simulink model "F16_nonlinear_simulation_R2018b"  (R2018b)
settings: Solver=VariableStepAuto  StartTime=0.0  StopTime=60  MaxStep=1.2  RelTol=1e-3
libraries: simulink x5, aerolibutil x2, aerolibanimutils x1, vrlib x1
settings Model: Creator=parth  LastModifiedBy=parth
settings DataIOCC: ReturnWorkspaceOutputs=on

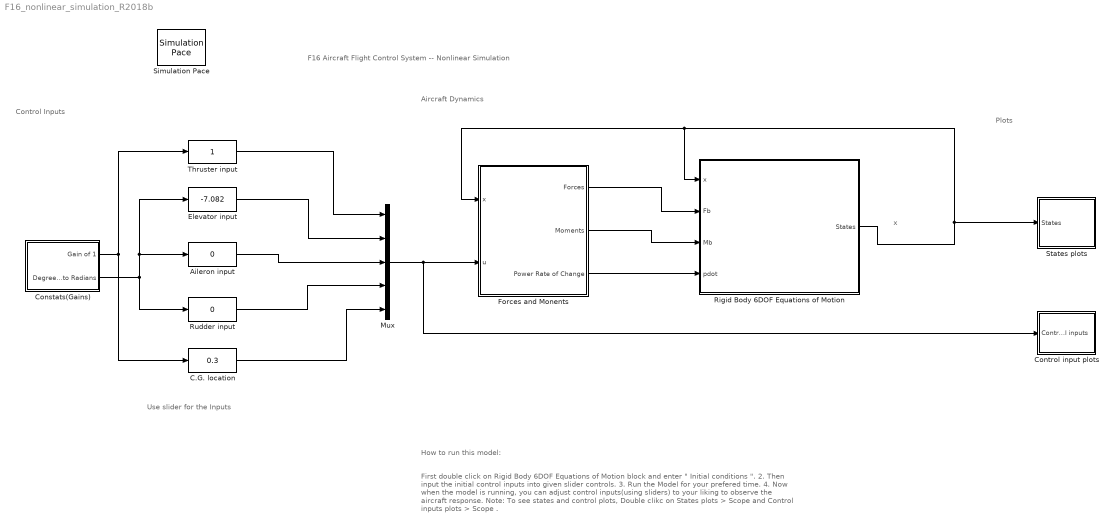
== system F16_nonlinear_simulation_R2018b ==
  note: x
  note: Plots
  note: Use slider for the Inputs
  note: F16 Aircraft Flight Control System -- Nonlinear Simulation
  note: Control Inputs
  note: Aircraft Dynamics
  note: First double click on Rigid Body 6DOF Equations of Motion block and enter " Initial conditions ".
      | 2. Then input the initial control inputs into given slider controls.
      | 3. Run the Model for your prefered time.
      | 4. Now when the model is running, you can adjust control inputs(using sliders) to your liking to observe the aircraft response.
      |
      | Note: To see states and control plots, Double clikc on States plots > Scope and Control inputs plots > Scope .
  note: How to run this model:
  Aileron input : simulink/Math Operations/Slider Gain  gain=0  low=-21.5  high=21.5
  C.G. location : simulink/Math Operations/Slider Gain  gain=0.3  low=0.3  high=0.4
  Constats(Gains) : Subsystem
  Control input plots : Subsystem
  Elevator input : simulink/Math Operations/Slider Gain  gain=-7.082  low=-25  high=25
  Forces and Monents : Subsystem
  Mux : Mux  Inputs=5
  "Rigid Body 6DOF Equations of Motion " : Subsystem  mask{V_init=502, alpha_init=0.3006, beta_init=0, p_init=0, q_init=0.3, r_init=0, phi_init=0, theta_init=0.3006, psi_init=0, Xe_init=0, Ye_init=0, h_init=1000, actual_power_init=90.566}
      mask prompts: V_init "V_init (ft/sec)"; alpha_init "alpha_init (rad)"; beta_init "beta_init (rad)"; p_init "p_init (rad/sec)"; q_init "q_init (rad/sec)"; r_init "r_init (rad/sec)"; phi_init "phi_init (rad)"; theta_init "theta_init (rad)"; psi_init "psi_init (rad)"; Xe_init "Xe_init (ft)"; Ye_init "Ye_init (ft)"; h_init "h_init (ft)"
      mask DialogControl ParameterGroupVar Prompt: Enter Aircraft Initial States here:
  Rudder input : simulink/Math Operations/Slider Gain  gain=0  low=-30  high=30
  Simulation Pace : aerolibanimutils/Simulation Pace  SimulationPace=1  SleepMode=Auto  OutputPaceError=off  SampleTime=1/30
  States plots : Subsystem
  Thruster input : simulink/Math Operations/Slider Gain  gain=1  low=0  high=1
  wires:
  Mux/1 -> Control input plots/1(Control inputs), Forces and Monents/2(u)
  Thruster input/1 -> Mux/1
  Elevator input/1 -> Mux/2
  Aileron input/1 -> Mux/3
  Forces and Monents/3(Power Rate of Change) -> "Rigid Body 6DOF Equations of Motion "/4(pdot)
  Constats(Gains)/1(Gain of 1) -> C.G. location/1, Thruster input/1
  Forces and Monents/1(Forces) -> "Rigid Body 6DOF Equations of Motion "/2(Fb)
  Forces and Monents/2(Moments) -> "Rigid Body 6DOF Equations of Motion "/3(Mb)
  Rudder input/1 -> Mux/4
  Constats(Gains)/2(Degree to Radians) -> Elevator input/1, Aileron input/1, Rudder input/1
  "Rigid Body 6DOF Equations of Motion "/1(States) -> Forces and Monents/1(x), "Rigid Body 6DOF Equations of Motion "/1(x), States plots/1(States)
  C.G. location/1 -> Mux/5

== system F16_nonlinear_simulation_R2018b/Constats(Gains) ==
  Constant(Gain) : Constant
  Degrees to Rad : Constant  Value=0.0175
  Gain of 1 : Outport
  Degree to Radians : Outport  Port=2
  wires:
  Degrees to Rad/1 -> Degree to Radians/1
  Constant(Gain)/1 -> Gain of 1/1

== system F16_nonlinear_simulation_R2018b/Control input plots ==
  Control inputs : Inport
  Demux : Demux
  Scope : Scope  NumInputPorts=4
  wires:
  Demux/4 -> Scope/4  "rudder"
  Demux/1 -> Scope/1  "throttle"
  Demux/3 -> Scope/3  "aileron"
  Control inputs/1 -> Demux/1
  Demux/2 -> Scope/2  "elevator"

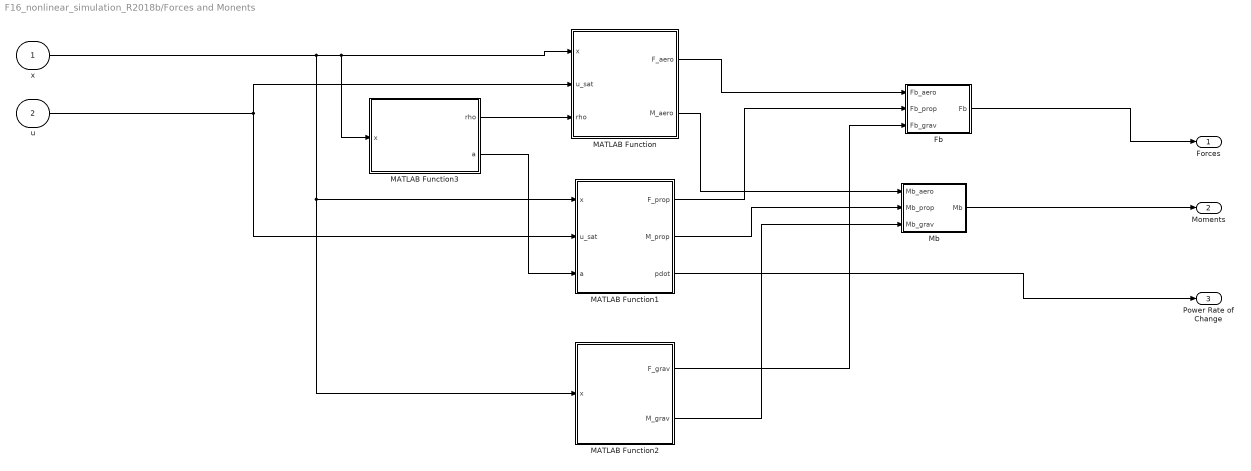
== system F16_nonlinear_simulation_R2018b/Forces and Monents ==
  x : Inport
  u : Inport  Port=2
  Fb : Subsystem
  MATLAB Function : MATLAB Function  TreatAsAtomicUnit=on
  MATLAB Function1 : MATLAB Function  TreatAsAtomicUnit=on
  MATLAB Function2 : MATLAB Function  TreatAsAtomicUnit=on
  MATLAB Function3 : MATLAB Function  TreatAsAtomicUnit=on
  Mb : Subsystem
  Forces : Outport
  Moments : Outport  Port=2
  Power Rate of Change : Outport  Port=3
  wires:
  Mb/1(Mb) -> Moments/1
  Fb/1(Fb) -> Forces/1
  x/1 -> MATLAB Function2/1(x), MATLAB Function1/1(x), MATLAB Function3/1(x), MATLAB Function/1(x)
  u/1 -> MATLAB Function1/2(u_sat), MATLAB Function/2(u_sat)
  MATLAB Function/1(F_aero) -> Fb/1(Fb_aero)
  MATLAB Function1/1(F_prop) -> Fb/2(Fb_prop)
  MATLAB Function2/1(F_grav) -> Fb/3(Fb_grav)
  MATLAB Function2/2(M_grav) -> Mb/3(Mb_grav)
  MATLAB Function1/2(M_prop) -> Mb/2(Mb_prop)
  MATLAB Function/2(M_aero) -> Mb/1(Mb_aero)
  MATLAB Function1/3(pdot) -> Power Rate of Change/1
  MATLAB Function3/1(rho) -> MATLAB Function/3(rho)
  MATLAB Function3/2(a) -> MATLAB Function1/3(a)

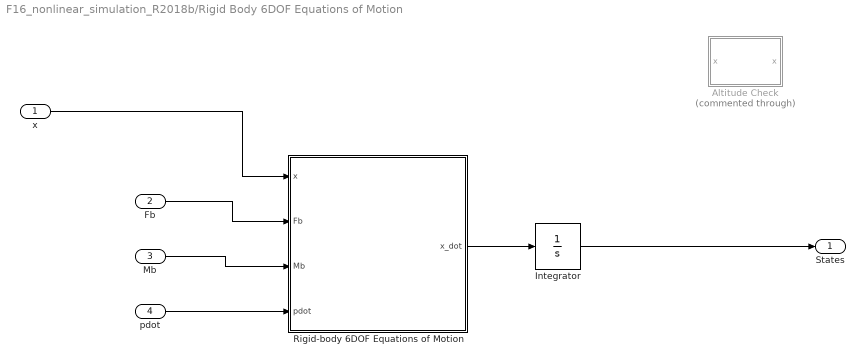
== system F16_nonlinear_simulation_R2018b/Rigid Body 6DOF Equations of Motion  ==
  x : Inport
  Fb : Inport  Port=2
  Mb : Inport  Port=3
  pdot : Inport  Port=4
  Altitude Check : MATLAB Function  Commented=through  TreatAsAtomicUnit=on
  Integrator : Integrator  InitialCondition=[(V_init*cos(alpha_init)*cos(beta_init)); (V_init*sin(beta_init)); (V_init*sin(alpha_init)*cos(beta_init)); p_init; q_init; r_init; phi_init; theta_init; psi_init; Xe_init; Ye_init; h_init; actual_power_init]
  Rigid-body 6DOF Equations of Motion : MATLAB Function  TreatAsAtomicUnit=on
  States : Outport
  wires:
  Fb/1 -> Rigid-body 6DOF Equations of Motion/2(Fb)
  x/1 -> Rigid-body 6DOF Equations of Motion/1(x)
  Rigid-body 6DOF Equations of Motion/1(x_dot) -> Integrator/1
  pdot/1 -> Rigid-body 6DOF Equations of Motion/4(pdot)
  Mb/1 -> Rigid-body 6DOF Equations of Motion/3(Mb)
  Integrator/1 -> States/1

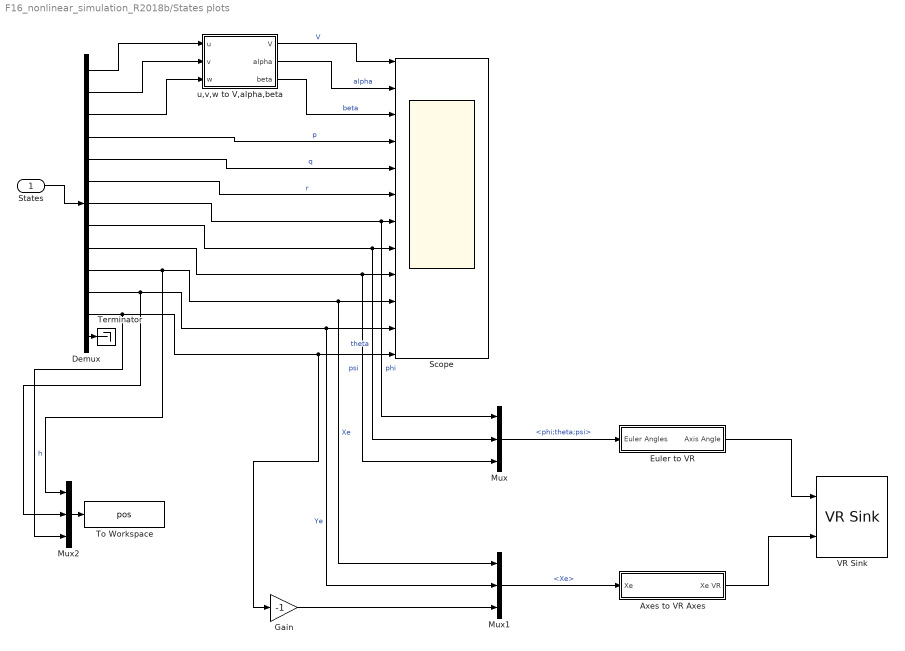
== system F16_nonlinear_simulation_R2018b/States plots ==
  States : Inport
  Axes to VR Axes : Subsystem
  Demux : Demux  Outputs=13
  Euler to VR : Subsystem
  Gain : Gain  Gain=-1
  Mux : Mux  Inputs=3
  Mux1 : Mux  Inputs=3
  Mux2 : Mux  Inputs=3
  Scope : Scope  NumInputPorts=12
  Terminator : Terminator
  To Workspace : ToWorkspace  VariableName=pos  SaveFormat=Timeseries  SampleTime=-1
  VR Sink : vrlib/VR Sink  InstantiateOnLoad=on  SampleTime=0.1  ViewEnable=on  RemoteChange=off  RemoteView=off  FieldsWritten=HL20.rotation.4.1.1.double#HL20.translation.3.1.1.double  WorldFileName=aeroblk_HL20.wrl  WorldDescription=aeroblk_HL20  AutoView=on  VideoDimensions=[]  AllowVariableSize=off  FigureProperties="{'Position', 'Name', 'Viewpoint', 'CameraBound', 'CameraDirection', 'CameraPosition', 'CameraUpVector', 'ZoomFactor', 'Antialiasing', 'Headlight', 'Lighting', 'NavPanel', 'Sound', 'StatusBar', 'Stereo3D', 'Stereo3DCameraOffset', 'Stereo3DHIT', 'ToolBar', 'Textures', 'Transparency', 'Triad', 'Wireframe', 'NavZones', 'NavMode', 'NavSpeed', 'CaptureFileFormat', 'CaptureFileName', 'Record2DCompressMethod', 'Record2DCompressQuality', 'Record2D', 'Record2DFileName', 'Record2DFPS'; [1.0000000000000000e+00   1.1800000000000000e+02   9.6000000000000000e+02   9.1100000000000000e+02], 'aeroblk_HL20', 'Rear Position', 'on', [-5.6194269145227393e-01  -1.3939411374335573e-04  -8.2717615541833223e-01], [1.4519874663616713e+02  -1.1012134985725118e-01   3.0148878051148063e+02], [4.0022421463915296e-03   9.9998782229421512e-01  -2.8874419604393194e-03], [1.0000000000000000e+00], 'on', 'on', 'on', 'halfbar', 'on', 'on', 'off', [1.0000000149011612e-01], [0.0000000000000000e+00], 'on', 'on', 'on', 'none', 'off', 'off', 'examine', 'normal', 'tif', '%f_anim_%n.tif', 'auto', [7.5000000000000000e+01], 'off', '%f_anim_%n.avi', 'auto'}"
  u,v,w to V,alpha,beta : MATLAB Function  TreatAsAtomicUnit=on
  wires:
  Demux/7 -> Mux/1, Scope/7  "phi"
  Demux/4 -> Scope/4  "p"
  Demux/13 -> Terminator/1
  Demux/1 -> u,v,w to V,alpha,beta/1(u)
  Demux/11 -> Mux2/2, Mux1/2, Scope/11  "Ye"
  Demux/3 -> u,v,w to V,alpha,beta/3(w)
  Demux/5 -> Scope/5  "q"
  States/1 -> Demux/1
  Demux/12 -> Mux2/3, Gain/1, Scope/12  "h"
  Demux/10 -> Mux2/1, Mux1/1, Scope/10  "Xe"
  Demux/2 -> u,v,w to V,alpha,beta/2(v)
  Demux/8 -> Mux/2, Scope/8  "theta"
  Demux/6 -> Scope/6  "r"
  Demux/9 -> Mux/3, Scope/9  "psi"
  u,v,w to V,alpha,beta/3(beta) -> Scope/3  "beta"
  u,v,w to V,alpha,beta/2(alpha) -> Scope/2  "alpha"
  u,v,w to V,alpha,beta/1(V) -> Scope/1  "V"
  Euler to VR/1(Axis Angle) -> VR Sink/1
  Mux/1 -> Euler to VR/1(Euler Angles)  "<phi;theta;psi>"
  Axes to VR Axes/1(Xe VR) -> VR Sink/2
  Mux1/1 -> Axes to VR Axes/1(Xe)  "<Xe>"
  Gain/1 -> Mux1/3
  Mux2/1 -> To Workspace/1

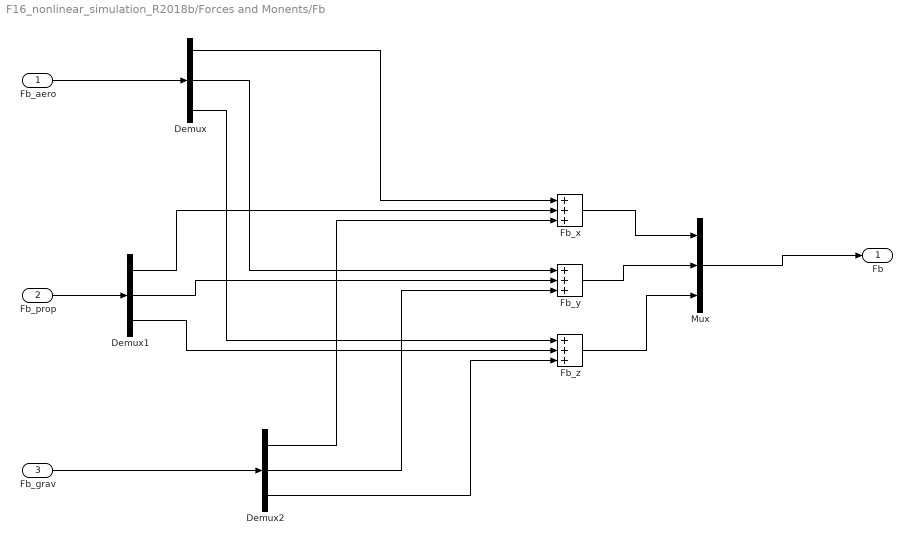
== system F16_nonlinear_simulation_R2018b/Forces and Monents/Fb ==
  Fb_aero : Inport
  Fb_prop : Inport  Port=2
  Fb_grav : Inport  Port=3
  Demux : Demux  Outputs=3
  Demux1 : Demux  Outputs=3
  Demux2 : Demux  Outputs=3
  Fb_x : Sum  Inputs=+++
  Fb_y : Sum  Inputs=+++
  Fb_z : Sum  Inputs=+++
  Mux : Mux  Inputs=3
  Fb : Outport
  wires:
  Demux1/2 -> Fb_y/2
  Demux/2 -> Fb_y/1
  Fb_x/1 -> Mux/1
  Demux/3 -> Fb_z/1
  Demux1/3 -> Fb_z/2
  Demux2/3 -> Fb_z/3
  Fb_z/1 -> Mux/3
  Demux1/1 -> Fb_x/2
  Demux2/1 -> Fb_x/3
  Fb_y/1 -> Mux/2
  Demux2/2 -> Fb_y/3
  Demux/1 -> Fb_x/1
  Mux/1 -> Fb/1
  Fb_aero/1 -> Demux/1
  Fb_prop/1 -> Demux1/1
  Fb_grav/1 -> Demux2/1

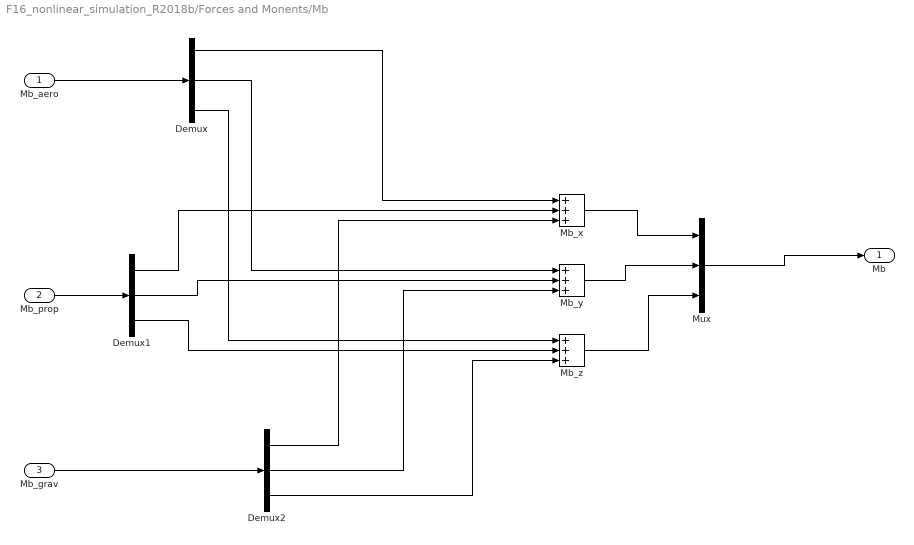
== system F16_nonlinear_simulation_R2018b/Forces and Monents/Mb ==
  Mb_aero : Inport
  Mb_prop : Inport  Port=2
  Mb_grav : Inport  Port=3
  Demux : Demux  Outputs=3
  Demux1 : Demux  Outputs=3
  Demux2 : Demux  Outputs=3
  Mb_x : Sum  Inputs=+++
  Mb_y : Sum  Inputs=+++
  Mb_z : Sum  Inputs=+++
  Mux : Mux  Inputs=3
  Mb : Outport
  wires:
  Demux1/2 -> Mb_y/2
  Demux/2 -> Mb_y/1
  Mb_x/1 -> Mux/1
  Demux/3 -> Mb_z/1
  Demux1/3 -> Mb_z/2
  Demux2/3 -> Mb_z/3
  Mb_z/1 -> Mux/3
  Demux1/1 -> Mb_x/2
  Demux2/1 -> Mb_x/3
  Mb_y/1 -> Mux/2
  Demux2/2 -> Mb_y/3
  Demux/1 -> Mb_x/1
  Mux/1 -> Mb/1
  Mb_aero/1 -> Demux/1
  Mb_prop/1 -> Demux1/1
  Mb_grav/1 -> Demux2/1

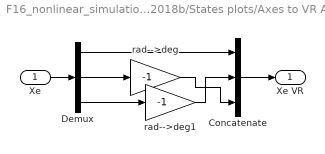
== system F16_nonlinear_simulation_R2018b/States plots/Axes to VR Axes ==
  Xe : Inport
  Concatenate : Concatenate  NumInputs=3
  Demux : Demux  Outputs=3
      settings: DisplayOption=none
  rad-->deg : Gain  Gain=-1  SaturateOnIntegerOverflow=on  OutDataTypeStr=Inherit: Same as input  ParamDataTypeStr=Inherit: Same as input
  rad-->deg1 : Gain  Gain=-1  SaturateOnIntegerOverflow=on  OutDataTypeStr=Inherit: Same as input  ParamDataTypeStr=Inherit: Same as input
  Xe VR : Outport  VectorParamsAs1DForOutWhenUnconnected=off
  wires:
  Xe/1 -> Demux/1
  Demux/1 -> Concatenate/1
  Demux/2 -> rad-->deg/1
  Demux/3 -> rad-->deg1/1
  Concatenate/1 -> Xe VR/1
  rad-->deg1/1 -> Concatenate/2
  rad-->deg/1 -> Concatenate/3

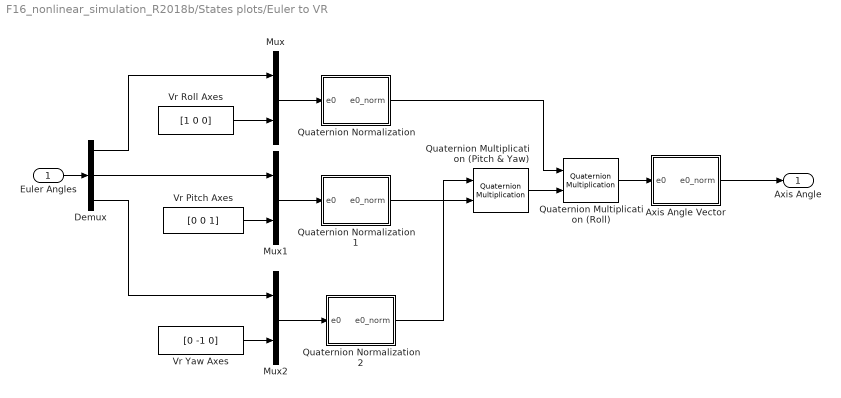
== system F16_nonlinear_simulation_R2018b/States plots/Euler to VR ==
  Euler Angles : Inport
  Axis Angle Vector : Subsystem
  Demux : Demux  Outputs=3
      settings: DisplayOption=none
  Mux : Mux  Inputs=2
  Mux1 : Mux  Inputs=2
  Mux2 : Mux  Inputs=2
  Quaternion Multiplication (Pitch & Yaw) : aerolibutil/Quaternion Multiplication
  Quaternion Multiplication (Roll) : aerolibutil/Quaternion Multiplication
  Quaternion Normalization : Subsystem
  Quaternion Normalization1 : Subsystem
  Quaternion Normalization2 : Subsystem
  Vr Pitch Axes : Constant  Value=[0 0 1]
  Vr Roll Axes : Constant  Value=[1 0 0]
  Vr Yaw Axes : Constant  Value=[0 -1 0]
  Axis Angle : Outport  VectorParamsAs1DForOutWhenUnconnected=off
  wires:
  Quaternion Multiplication (Roll)/1 -> Axis Angle Vector/1(e0)
  Quaternion Multiplication (Pitch & Yaw)/1 -> Quaternion Multiplication (Roll)/2
  Axis Angle Vector/1(e0_norm) -> Axis Angle/1
  Quaternion Normalization/1(e0_norm) -> Quaternion Multiplication (Roll)/1
  Quaternion Normalization2/1(e0_norm) -> Quaternion Multiplication (Pitch & Yaw)/1
  Quaternion Normalization1/1(e0_norm) -> Quaternion Multiplication (Pitch & Yaw)/2
  Mux2/1 -> Quaternion Normalization2/1(e0)
  Mux1/1 -> Quaternion Normalization1/1(e0)
  Mux/1 -> Quaternion Normalization/1(e0)
  Demux/3 -> Mux2/1
  Vr Yaw Axes/1 -> Mux2/2
  Demux/2 -> Mux1/1
  Vr Pitch Axes/1 -> Mux1/2
  Demux/1 -> Mux/1
  Vr Roll Axes/1 -> Mux/2
  Euler Angles/1 -> Demux/1

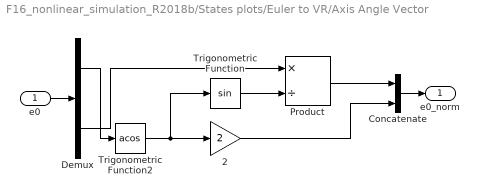
== system F16_nonlinear_simulation_R2018b/States plots/Euler to VR/Axis Angle Vector ==
  e0 : Inport
  2 : Gain  Gain=2  SaturateOnIntegerOverflow=on  OutDataTypeStr=Inherit: Same as input  ParamDataTypeStr=Inherit: Same as input
  Concatenate : Concatenate
  Demux : Demux  Outputs=[1 3 ]
      settings: DisplayOption=none
  Product : Product  Inputs=*/  InputSameDT=on  SaturateOnIntegerOverflow=on  OutDataTypeStr=Inherit: Same as first input
  Trigonometric Function : Trigonometry
  Trigonometric Function2 : Trigonometry  Operator=acos
  e0_norm : Outport  VectorParamsAs1DForOutWhenUnconnected=off
  wires:
  Demux/1 -> Trigonometric Function2/1
  Demux/2 -> Product/1
  Concatenate/1 -> e0_norm/1
  Product/1 -> Concatenate/1
  2/1 -> Concatenate/2
  Trigonometric Function/1 -> Product/2
  Trigonometric Function2/1 -> Trigonometric Function/1, 2/1
  e0/1 -> Demux/1

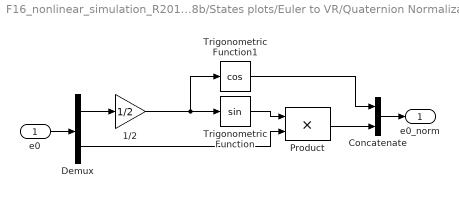
== system F16_nonlinear_simulation_R2018b/States plots/Euler to VR/Quaternion Normalization ==
  e0 : Inport
  1/2 : Gain  Gain=1/2  SaturateOnIntegerOverflow=on  OutDataTypeStr=Inherit: Same as input  ParamDataTypeStr=Inherit: Same as input
  Concatenate : Concatenate
  Demux : Demux  Outputs=[1 3]
      settings: DisplayOption=none
  Product : Product  InputSameDT=on  SaturateOnIntegerOverflow=on  OutDataTypeStr=Inherit: Same as first input
  Trigonometric Function : Trigonometry
  Trigonometric Function1 : Trigonometry  Operator=cos
  e0_norm : Outport  VectorParamsAs1DForOutWhenUnconnected=off
  wires:
  Trigonometric Function1/1 -> Concatenate/1
  Demux/2 -> Product/2
  Demux/1 -> 1/2/1
  Concatenate/1 -> e0_norm/1
  Product/1 -> Concatenate/2
  Trigonometric Function/1 -> Product/1
  1/2/1 -> Trigonometric Function1/1, Trigonometric Function/1
  e0/1 -> Demux/1

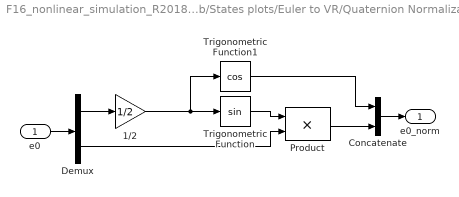
== system F16_nonlinear_simulation_R2018b/States plots/Euler to VR/Quaternion Normalization1 ==
  e0 : Inport
  1/2 : Gain  Gain=1/2  SaturateOnIntegerOverflow=on  OutDataTypeStr=Inherit: Same as input  ParamDataTypeStr=Inherit: Same as input
  Concatenate : Concatenate
  Demux : Demux  Outputs=[1 3]
      settings: DisplayOption=none
  Product : Product  InputSameDT=on  SaturateOnIntegerOverflow=on  OutDataTypeStr=Inherit: Same as first input
  Trigonometric Function : Trigonometry
  Trigonometric Function1 : Trigonometry  Operator=cos
  e0_norm : Outport  VectorParamsAs1DForOutWhenUnconnected=off
  wires:
  e0/1 -> Demux/1
  1/2/1 -> Trigonometric Function/1, Trigonometric Function1/1
  Trigonometric Function/1 -> Product/1
  Product/1 -> Concatenate/2
  Concatenate/1 -> e0_norm/1
  Demux/1 -> 1/2/1
  Demux/2 -> Product/2
  Trigonometric Function1/1 -> Concatenate/1

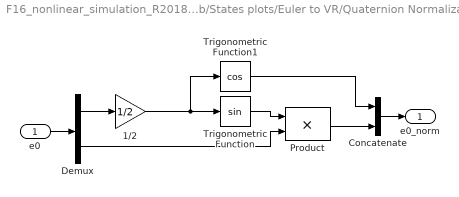
== system F16_nonlinear_simulation_R2018b/States plots/Euler to VR/Quaternion Normalization2 ==
  e0 : Inport
  1/2 : Gain  Gain=1/2  SaturateOnIntegerOverflow=on  OutDataTypeStr=Inherit: Same as input  ParamDataTypeStr=Inherit: Same as input
  Concatenate : Concatenate
  Demux : Demux  Outputs=[1 3]
      settings: DisplayOption=none
  Product : Product  InputSameDT=on  SaturateOnIntegerOverflow=on  OutDataTypeStr=Inherit: Same as first input
  Trigonometric Function : Trigonometry
  Trigonometric Function1 : Trigonometry  Operator=cos
  e0_norm : Outport  VectorParamsAs1DForOutWhenUnconnected=off
  wires:
  Trigonometric Function1/1 -> Concatenate/1
  Demux/2 -> Product/2
  Demux/1 -> 1/2/1
  Concatenate/1 -> e0_norm/1
  Product/1 -> Concatenate/2
  Trigonometric Function/1 -> Product/1
  1/2/1 -> Trigonometric Function1/1, Trigonometric Function/1
  e0/1 -> Demux/1

== matlab function F16_nonlinear_simulation_R2018b/Forces and Monents/MATLAB Function1 ==
  data: x input; F_prop output; u_sat input; M_prop output; pdot output; a input
function [F_prop, M_prop, pdot] = F16_propulsion(x,u_sat,a)
%Calculate Propulsive Forces and Moments 
% u_sat = [delta_T, delta_e, delta_a, delta_r]
%
% based on work for Stanle Bak
% https://github.com/stanleybak/AeroBenchVVPython

%% TGEAR function
% convert command [0,1] to commanded power [0,100]
if (u_sat(1) <= .77)
    comm_power = 64.94 * u_sat(1);  % commanded power
else
    comm_power = 217.38 * u_sat(1) - 117.38;
end

%% RTAU function
% time constant for first order lag in engine power dynamic repsonse
    function rt = rtau(delta_power)
        if(delta_power <= 25)
            rt = 1.0;
        elseif(delta_power >= 50)
            rt = .1;
        else
            rt = 1.9 - .036*delta_power;
        end
    end
    
%% PDOT function
% comptute rate of change power fromm given actual power and commanded
% power
if(comm_power >= 50)
    if(x(13) >= 50)
        t = 5;
        p2 = comm_power;
    else
        p2 = 60;
        t = rtau(p2 - x(13));
    end
else
    if (x(13) >= 50)
        t = 5;
        p2 = 40;
    else
        p2 = comm_power;
        t = rtau(p2 - x(13));
    end
end

pdot = t * (p2 - x(13));

%% THRUST function
% calculate engine thrust
V = sqrt(x(1)^2 + x(2)^2 + x(3)^2);
M = V/a; % mach number

a = [1060,670,880,1140,1500,1860;...
    635,425,690,1010,1330,1700;...
    60,25,345,755,1130,1525;...
    -1020,-170,-300,350,910,1360;...
    -2700,-1900,-1300,-247,600,1100;...
    -3600,-1400,-595,-342,-200,700]';

b = [12680,9150,6200,3950,2450,1400;...
    12680,9150,6313,4040,2470,1400;...
    12610,9312,6610,4290,2600,1560;...
    12640,9839,7090,4660,2840,1660;...
    12390,10176,7750,5320,3250,1930;...
    11680,9848,8050,6100,3800,2310;]';

c = [20000,15000,10800,7000,4000,2500;...
    21420,15700,11225,7323,4435,2600;...
    22700,16860,12250,8154,5000,2835;...
    24240,18910,13760,9285,5700,3215;...
    26070,21075,15975,11115,6860,3950;...
    28886,23319,18300,13484,8642,5057]';

if (x(12)<0)
    x(12) = 0.01;
end

h =.0001 * x(12);
i = fix(h);  
if(i >= 5)
    i = 4;
end

dh = h - i;
rm = 5 * M;
m = fix(rm);
if(m >= 5)
    m = 4;
end

dm = rm - m;
cdh = 1 - dh;

i = i + 1;
m = m + 1;

s = b(i, m) * cdh + b(i + 1, m) * dh;
t = b(i, m + 1) * cdh + b(i + 1, m + 1) * dh;
tmil = s + (t - s) * dm;

if (x(13) < 50)
    s = a(i, m) * cdh + a(i + 1, m) * dh;
    t = a(i, m + 1) * cdh + a(i + 1, m + 1) * dh;
    tidl = s + (t - s) * dm;
    thrust = tidl + (tmil - tidl) * x(13) * .02;
else 
    s = c(i, m) * cdh + c(i + 1, m) * dh;
    t = c(i, m + 1) * cdh + c(i + 1, m + 1) * dh;
    tmax = s + (t - s) * dm;
    thrust = tmil + (tmax - tmil) * (x(13) - 50) * .02;
end


%% Propulsive Force and Moment about body axis
F_prop = [thrust; 0; 0];
M_prop = [0; 0; 0];
end

== matlab function F16_nonlinear_simulation_R2018b/Forces and Monents/MATLAB Function ==
  data: x input; F_aero output; u_sat input; M_aero output; rho input
function [F_aero, M_aero] = F16_aerodynamics(x,u_sat,rho)
% Compute F16 Body-axis Aerodynamics forces and moments
% u_sat = [delta_T, delta_e, delta_a, delta_r, x_cg]
%
% Arodynamic model for F16 in form of Polynomial function
% is used here instead of data tables as described in [1]
%
% Ref:
% [1] GLOBAL NONLINEAR PARAMETRIC MODELING WITH APPLICATION TO 
%     F-16 AERODYNAMICS, by Eugene A. Morelli.

% physical parameters
% Ref: Aircraft Control and Simulation, Stevens & Lewis.
S = 300; % wing area, ft^2
c_bar = 11.32; % mean aero cord, ft
b = 30; % wing span, ft
xcg_ref = 0.35;%*c_bar; % reference c.g. location
x_cg = u_sat(5);%*c_bar; % c.g. location % VARIABLE % Fixed here

% convert body-axis velocity to (alpha,beta,V)
V = sqrt(x(1)^2 + x(2)^2 + x(3)^2); % m/sec
alpha = atan(x(3)/x(1)); % rad
beta = asin(x(2)/V); % rad

% variable ranges  % bound
%    -- Table 1 [1]
 if alpha < -0.1745      % -10 to 45 deg
    alpha = -0.1745;
elseif alpha > 0.7854
    alpha = 0.7854;
end
if beta < -0.5236       % -30 to 30 deg
    beta = -0.5236;
elseif beta > 0.5236
    beta = 0.5236;
end

% aerodynamic polynomial model
%    -- Table 2 [1]
Cx_0 = -1.943367e-02 + 2.136104e-01*alpha - 2.903457e-01*(u_sat(2)^2) ...
       -3.348641e-03*u_sat(2) - 2.060504e-01*alpha*u_sat(2) + ...
       6.988016e-01*(alpha^2) - 9.035381e-01*(alpha^3);
Cx_q = 4.833383e-01 + 8.644627e+00*alpha + 1.131098e+01*(alpha^2) ...
       - 7.422961e+01*(alpha^3) + 6.075776e+01*(alpha^4);
Cy_0 = -1.145916e+00*beta + 6.016057e-02*u_sat(3) + 1.642479e-01*u_sat(4);
Cy_p = -1.006733e-01 + 8.679799e-01*alpha + 4.260586e+00*(alpha^2) ...
       - 6.923267e+00*(alpha^3);
Cy_r = 8.071648e-01 + 1.189633e-01*alpha + 4.177702e+00*(alpha^2) ...
       - 9.162236e+00*(alpha^3);
Cz_0 = (1-(beta^2))*(-1.378278e-01 - 4.211369e+00*alpha + ...
        4.775187e+00*(alpha^2) - 1.026225e+01*(alpha^3) + ...
        8.399763e+00*(alpha^4)) - 4.354000e-01*u_sat(2);
Cz_q = -3.054956e+01 - 4.132305e+01*alpha + 3.292788e+02*(alpha^2) ...
       - 6.848038e+02*(alpha^3) + 4.080244e+02*(alpha^4);
Cl_0 = -1.058583e-01*beta - 5.776677e-01*alpha*beta - ...
       1.672435e-02*(alpha^2)*beta + 1.357256e-01*(beta^2) ...
       + 2.172952e-01*alpha*(beta^2) + 3.464156e+00*(alpha^3)*beta ...
       - 2.835451e+00*(alpha^4)*beta - 1.098104e+00*(alpha^2)*(beta^2);
Cl_p = -4.126806e-01 - 1.189974e-01*alpha + 1.247721e+00*(alpha^2) ...
       - 7.391132e-01*(alpha^3);
Cl_r = 6.250437e-02 + 6.067723e-01*alpha - 1.101964e+00*(alpha^2) ...
       + 9.100087e+00*(alpha^3) - 1.192672e+01*(alpha^4);
Cl_delta_a = -1.463144e-01 - 4.073901e-02*alpha + 3.253159e-02*beta ...
             + 4.851209e-01*(alpha^2) + 2.978850e-01*alpha*beta ...
             - 3.746393e-01*(alpha^2)*beta - 3.213068e-01*(alpha^3);
Cl_delta_r = 2.635729e-2 - 2.192910e-02*alpha - 3.152901e-03*beta ...
             - 5.817803e-02*alpha*beta + 4.516159e-01*(alpha^2)*beta ...
             - 4.928702e-01*(alpha^3)*beta - 1.579864e-02*(beta^2);
Cm_0 = -2.029370e-02 + 4.660702e-02*alpha - 6.012308e-01*u_sat(2) ...
       -8.062977e-02*alpha*u_sat(2) + 8.320429e-02*(u_sat(2)^2) + ...
       5.018538e-01*(alpha^2)*u_sat(2) + 6.378864e-01*(u_sat(2)^3) ...
       + 4.226356e-01*alpha*(u_sat(2)^2);
Cm_q = -5.159153e+00 - 3.554716e+00*alpha - 3.598636e+01*(alpha^2) + ...
       2.247355e+02*(alpha^3) - 4.120991e+02*(alpha^4) ...
       + 2.411750e+02*(alpha^5);
Cn_0 = 2.993363e-01*beta + 6.594004e-02*alpha*beta - ...
       2.003125e-01*(beta^2) - 6.233977e-02*alpha*(beta^2) ...
       - 2.107885e+00*(alpha^2)*beta + 2.141420e+00*(alpha^2)*(beta^2) ...
       + 8.476901e-01*(alpha^3)*beta;
Cn_p = 2.677652e-02 - 3.298246e-01*alpha + 1.926178e-01*(alpha^2) ...
       + 4.013325e+00*(alpha^3) - 4.404302e+00*(alpha^4);
Cn_r = -3.698756e-01 - 1.167551e-01*alpha - 7.641297e-01*(alpha^2);
Cn_delta_a = -3.348717e-02 + 4.276655e-02*alpha + 6.573646e-03*beta ... 
             + 3.535831e-01*alpha*beta - 1.373308e+00*(alpha^2)*beta ...
             + 1.237582e+00*(alpha^3)*beta + 2.302543e-01*(alpha^2) ...
             - 2.512876e-01*(alpha^3) + 1.588105e-01*(beta^3) ...
             - 5.199526e-01*alpha*(beta^3);
Cn_delta_r = -8.115894e-02 - 1.156580e-02*alpha + 2.514167e-02*beta ...
             + 2.038748e-01*alpha*beta - 3.337476e-01*(alpha^2)*beta ... 
             + 1.004297e-01*(alpha^2);
   
% dynamic pressure
q_bar = 0.5*rho*V*V;

% non-dimensional
p_nd = 0.5*x(4)*b/V;
q_nd = 0.5*x(5)*c_bar/V;
r_nd = 0.5*x(6)*b/V;

% aerodynamic forces
Cx = Cx_0 + q_nd*Cx_q;
Cy = Cy_0 + p_nd*Cy_p + r_nd*Cy_r;
Cz = Cz_0 + q_nd*Cz_q;

% aerodynamic moments
Cl = Cl_0 + p_nd*Cl_p + r_nd*Cl_r + u_sat(3)*Cl_delta_a + ...
        u_sat(4)*Cl_delta_r;
Cm = Cm_0 + q_nd*Cm_q + Cz*(xcg_ref - x_cg);
Cn = Cn_0 + p_nd*Cn_p + r_nd*Cn_r + u_sat(3)*Cn_delta_a + ...
        u_sat(4)*Cn_delta_r - Cy*c_bar*(xcg_ref - x_cg)/b;
    
F_aero = q_bar*S*[Cx; Cy; Cz];
M_aero = q_bar*S*[Cl*b; Cm*c_bar; Cn*b];
end

== matlab function F16_nonlinear_simulation_R2018b/Forces and Monents/MATLAB Function2 ==
  data: x input; F_grav output; M_grav output
function [F_grav, M_grav] = gravity_model(x)
% Gravity forces and moments in body axis system
% 
% References : Ch. 7, Aircraft Flight Dynamics and Control,
%               by Wayne Durham.

g = 32.17; %ft/s^2
F_grav = g*[-sin(x(8)); sin(x(7))*cos(x(8)); cos(x(7))*cos(x(8))];
M_grav = [0; 0; 0];
end

== matlab function F16_nonlinear_simulation_R2018b/Rigid Body 6DOF Equations of Motion /Rigid-body 6DOF Equations of Motion ==
  data: x input; x_dot output; Fb input; Mb input; pdot input
function x_dot = nonlinear_6DOF(x, Fb, Mb, pdot)
% rigid body aircraft 6DOF nonlinear equations of motion
% in Body-axis with Flat Earth Assumption.
% x = [u,v,w,p,q,r,phi,theta,psi,xe,ye,h(=ze)), pdot]  ==> must be (13,1)
%%%% u = [delta_T, delta_e, delta_a, delta_r]

% u,v,w -> in m/s
% p,q,r -> in rad/sec
% phi,theta,psi -> rad
% xe,ye,h -> m
%%%% delta_T -> between 0 to 1
%%%% delta_e, delta_a, delta_r -> deg

% References : Ch. 7, Aircraft Flight Dynamics and Control,
%               by Wayne Durham.

% physical parameters
% Ref: Aircraft Control and Simulation, Stevens & Lewis.
m = 637.2397; %20500/32.17; % lbs

% inertia matrix    % slug*ft^2    
Ib = [9496, 0.0, -982;
    0.0, 55814, 0.0;
    -982, 0.0, 63100];

% inverse inertia matrix
% precomputed for faster executions
Ib_inv =    1.0e-03 * [
    0.1055         0    0.0016;
         0    0.0179         0;
    0.0016         0    0.0159;
];


% to speed up the calcultions
s_phi = sin(x(7));
c_phi = cos(x(7));
s_theta = sin(x(8));
c_theta = cos(x(8));
t_theta = tan(x(8));
s_psi = sin(x(9));
c_psi = cos(x(9));

% W-x matrix
omega_b = [0 -x(6) x(5); ...
         x(6) 0 -x(4); ...
         -x(5) x(4) 0];

% local horizontal(H) frame to body(B) frame
T_BH = [1 s_phi*t_theta c_phi*t_theta;
      0 c_phi -s_phi;
      0 s_phi/c_theta c_phi/c_theta];

% Body(B) frame to Earth-fixed(E) frame
T_EB = [c_theta*c_psi, -c_phi*s_psi + s_phi*s_theta*c_psi, ... 
                                  s_phi*s_psi + c_phi*s_theta*c_psi; ...
      c_theta*s_psi, c_phi*c_psi + s_phi*s_theta*s_psi, ...
                                  -s_phi*c_psi + c_phi*s_theta*s_psi; ...
      s_theta, -s_phi*c_theta, -c_phi*c_theta;
];

%% Equations of Motion (Body axis)
x_dot = zeros(13,1);
x_dot(1:3,1) =  (Fb/m) - omega_b*x(1:3,1);
x_dot(4:6,1) = Ib_inv*(Mb - omega_b*Ib*x(4:6,1));
x_dot(7:9,1) =  T_BH*x(4:6,1);
x_dot(10:12,1) = T_EB*x(1:3,1);
x_dot(13,1) = pdot;
end

== matlab function F16_nonlinear_simulation_R2018b/Forces and Monents/MATLAB Function3 ==
  data: x input; rho output; a output
function [rho, a] = atmospheric_model(x)
% calculate the atmospheric density(in Kg/m^3) and speed of sound
% at the given altitude
% 
% Ref: Stevens & Lewis, "Aircraft Control and Simulation"
    altitude = x(12);
    ro = 2.377e-3;
    tfac = 1 - .703e-5 * altitude;

    if altitude >= 35000 % in stratosphere
        t = 390;
    else
        t = 519 * tfac; % 3 rankine per atmosphere (3 rankine per 1000 ft)
    end
    rho = ro * tfac^4.14;

    %speed of sound
    a = sqrt(1.4 * 1716.3 * t);
end

== matlab function F16_nonlinear_simulation_R2018b/Rigid Body 6DOF Equations of Motion /Altitude Check ==
  data: x input; x output
function x = fcn(x)

% Altitude check
if (x(12) <= 0.01)
    x(12) = 0.01;
end

end

== matlab function F16_nonlinear_simulation_R2018b/States plots/u,v,w to V,alpha,beta ==
  data: u input; V output; v input; w input; alpha output; beta output
function [V,alpha,beta] = fcn(u,v,w)

V = sqrt(u^2 + v^2 + w^2);
alpha = atan(w/u);
beta = asin(v/V);

end
